simulink model "mls_driver_nasz"  (R2023a)
settings: Solver=ode5  StartTime=0.0  StopTime=inf  FixedStep=0.001  RelTol=1e-3  AbsTol=1e-6
InitFcn:
  | load ml_sensor
undefined symbols (not defined in the file or in its folder): RTDAC4PCIBaseAddress
settings Model: SimulationMode=external  ExtModeEnableFloating=off  ExtModeTrigDuration=40000  ExtModeTrigDirection=either  ExtModeArchiveFileName=exp01.mat  ExtModeArchiveDirName=h:\temp  ExtModeWriteAllDataToWs=on  Creator=Adam Pilat  LastModifiedBy=HP
settings SolverCC: AutoScaleAbsTol=off  AlgebraicLoopSolver=TrustRegion
settings DataIOCC: ExternalInput=[]  InitialState=[]  MaxDataPoints=5000  SaveFormat=Array  SignalLoggingSaveFormat=ModelDataLogs  SaveOutput=off  SaveTime=off  ReturnWorkspaceOutputs=off  SignalLoggingName=sigsOut
settings OptimizationCC: BooleanDataType=off  ExpressionDepthLimit=2147483647  InitFltsAndDblsToZero=on  LifeSpan=inf
settings DebuggingCC: SaveWithParameterizedLinksMsg=none  UnderspecifiedInitializationDetection=Classic  MergeDetectMultiDrivingBlocksExec=none  SignalResolutionControl=TryResolveAllWithWarning  MultiTaskDSMMsg=warning  MultiTaskCondExecSysMsg=none  IntegerOverflowMsg=none  FcnCallInpInsideContextMsg=warning  UnconnectedInputMsg=warning  UnconnectedOutputMsg=warning  UnconnectedLineMsg=warning  StateNameClashWarn=warning  SFUnexpectedBacktrackingDiag=warning  SFNoUnconditionalDefaultTransitionDiag=warning  SFExecutionAtInitializationDiag=none  IntegerSaturationMsg=none  ArithmeticOperatorsInVariantConditions=warning
settings HardwareCC: ProdBitPerLong=64  ProdLargestAtomicFloat=None  ProdHWDeviceType=Intel->x86-64  TargetBitPerLong=64  TargetBitPerPointer=64  TargetIntDivRoundTo=Zero  TargetEndianess=LittleEndian  TargetWordSize=64  TargetHWDeviceType=Intel->x86-64
settings ModelReferenceCC: PropagateSignalLabelsOutOfModel=off
settings SFSimCC: SimUseLocalCustomCode=off  CustomCodeUndefinedFunction=UseInterfaceOnly
settings RTWCC: Description=Real-Time Windows Target  SystemTargetFile=rtwin.tlc  TemplateMakefile=rtwin.tmf  RTWUseLocalCustomCode=off
settings CodeAppCC: StateflowObjectComments=on
settings RTWinTargetCC: TargetFcnLib=ansi_tfl_tmw.mat  TargetPreCompLibLocation=C:\Program Files\MATLAB\R2015aSP1\toolbox\sldrt\lib\win64  MultiwordTypeDef=System defined  DynamicStringBufferSize=256  ModelReferenceCompliant=off  CompOptLevelCompliant=off  GroupInternalDataByFunction=off  RemoveDisableFunc=off  RemoveResetFunc=off  MDXCompliant=off  UseToolchainInfoCompliant=off  CoderGroups=[]  AccessMethods=[]  LookupTableObjectStructAxisOrder=1,2,3,4,...  LUTObjectStructOrderExplicitValues=Size,Breakpoints,Table  LUTObjectStructOrderEvenSpacing=Size,Breakpoints,Table  ArrayLayout=Column-major  UnsupportedSFcnMsg=error  ERTHeaderFileRootName=$R$E  ERTSourceFileRootName=$R$E  ERTDataFileRootName=$R_data  OptimizeReductions=off
settings ConfigComp: CovMetricSettings=dw  CovSaveCumulativeToWorkspaceVar=on  CovSaveSingleToWorkspaceVar=on  CovExternalEMLEnable=off  CovSFcnEnable=off

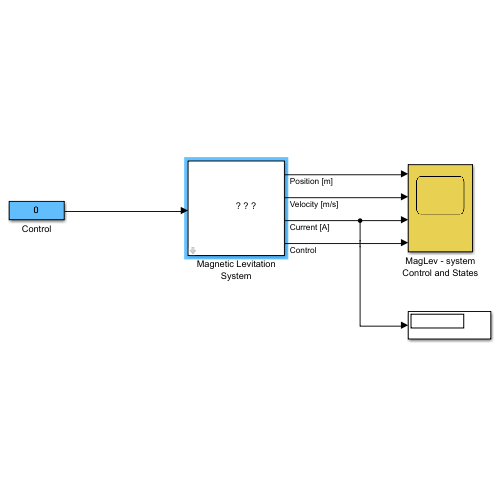
[thumbnail: Simulink's stored preview of the top-level diagram]
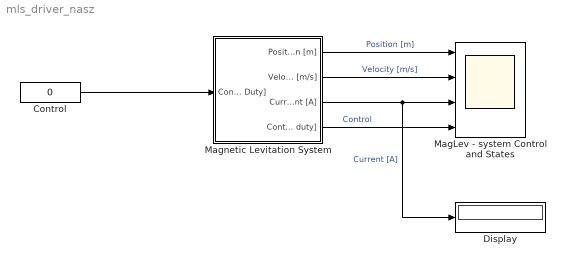
== system mls_driver_nasz ==
  Control : Constant  Value=0
  Display : Display
  MagLev - system Control and States : Scope  NumInputPorts=4
  Magnetic Levitation System : Subsystem  mask(Magnetic Levitation 1 - System){BA=RTDAC4PCIBaseAddress, T0=0.001}
      mask prompts: BA "Base Address (dec):"; T0 "Sampling period [s]:"
      mask help:
      | MagLev1 - System connection for the real-time operating mode
      | (c) InTeCo 2005
      mask Display: image(imread('MagLev1.tif'))
  wires:
  Magnetic Levitation System/1(Position [m]) -> MagLev - system Control and States/1  "Position [m]"
  Magnetic Levitation System/2(Velocity [m/s]) -> MagLev - system Control and States/2  "Velocity [m/s]"
  Magnetic Levitation System/3(Current [A]) -> Display/1, MagLev - system Control and States/3  "Current [A]"
  Magnetic Levitation System/4(Control [PWM duty]) -> MagLev - system Control and States/4  "Control"
  Control/1 -> Magnetic Levitation System/1(Control [PWM Duty])

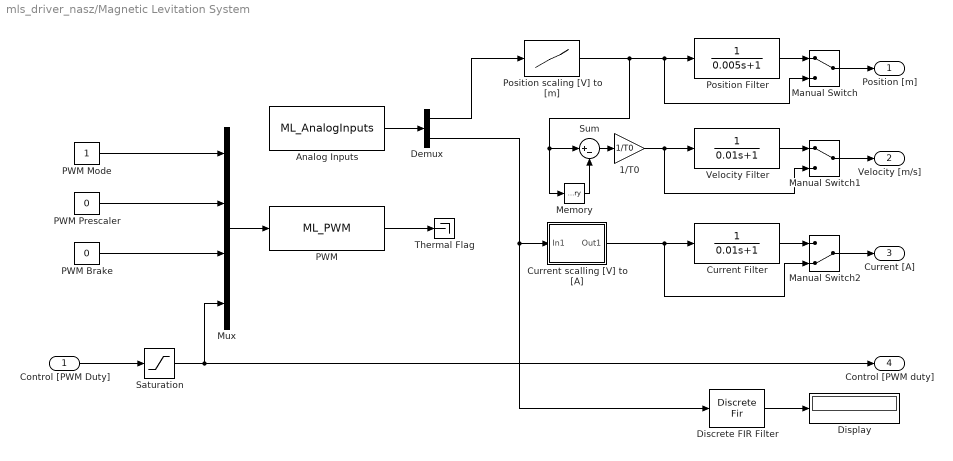
== system mls_driver_nasz/Magnetic Levitation System ==
  Control [PWM Duty] : Inport
  1/T0 : Gain  Gain=1/T0  SaturateOnIntegerOverflow=on  OutDataTypeStr=Inherit: Same as input  ParamDataTypeStr=Inherit: Same as input
  Analog Inputs : S-Function  FunctionName=ML_AnalogInputs  Parameters=BA, [4 2], [1 1], T0  SFunctionDeploymentMode=off  EnableBusSupport=off
  Current Filter : TransferFcn  Denominator=[0.01 1]
  Current scalling [V] to [A] : Subsystem
      mask Display: plot([0    0.5000    1.0000    1.5000    2.0000    2.5000], [-0.0317    0.4951    1.0302    1.5738    2.1258    2.6863]);
  Demux : Demux  Outputs=2
      settings: DisplayOption=none
  Discrete FIR Filter : DiscreteFir  Coefficients=ones(1,1000)/1000
  Display : Display
  Manual Switch : ManualSwitch
  Manual Switch1 : ManualSwitch
  Manual Switch2 : ManualSwitch  CurrentSetting=0
  Memory : Memory
  Mux : Mux
  PWM : S-Function  FunctionName=ML_PWM  Parameters=BA, T0  SFunctionDeploymentMode=off  EnableBusSupport=off
  PWM Brake : Constant  Value=0
  PWM Mode : Constant
  PWM Prescaler : Constant  Value=0
  Position Filter : TransferFcn  Denominator=[0.005 1]
  Position scaling [V] to [m] : Lookup  InputValues=SensorData.Sensor_V(end:-1:1)  Table=SensorData.Distance_m(end:-1:1)
  Saturation : Saturate  UpperLimit=1  LowerLimit=0
  Sum : Sum  Inputs=|+-  InputSameDT=on  SaturateOnIntegerOverflow=on  OutDataTypeStr=Inherit: Same as first input
  Thermal Flag : Terminator
  Velocity Filter : TransferFcn  Denominator=[0.01 1]
  Position [m] : Outport
  Velocity [m/s] : Outport  Port=2
  Current [A] : Outport  Port=3
  Control [PWM duty] : Outport  Port=4
  wires:
  Manual Switch1/1 -> Velocity [m/s]/1
  Current Filter/1 -> Manual Switch2/1
  Velocity Filter/1 -> Manual Switch1/1
  Position Filter/1 -> Manual Switch/1
  Demux/1 -> Position scaling [V] to [m]/1
  Demux/2 -> Discrete FIR Filter/1, Current scalling [V] to [A]/1(In1)
  Current scalling [V] to [A]/1(Out1) -> Manual Switch2/2, Current Filter/1
  1/T0/1 -> Manual Switch1/2, Velocity Filter/1
  Sum/1 -> 1/T0/1
  Memory/1 -> Sum/2
  Analog Inputs/1 -> Demux/1
  Mux/1 -> PWM/1
  PWM Prescaler/1 -> Mux/2
  PWM Mode/1 -> Mux/1
  PWM/1 -> Thermal Flag/1
  Saturation/1 -> Mux/4, Control [PWM duty]/1
  Control [PWM Duty]/1 -> Saturation/1
  Manual Switch2/1 -> Current [A]/1
  PWM Brake/1 -> Mux/3
  Position scaling [V] to [m]/1 -> Manual Switch/2, Position Filter/1, Memory/1, Sum/1
  Manual Switch/1 -> Position [m]/1
  Discrete FIR Filter/1 -> Display/1

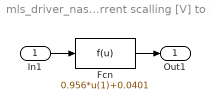
== system mls_driver_nasz/Magnetic Levitation System/Current scalling [V] to [A] ==
  In1 : Inport
  Fcn : Fcn  Expr=0.956*u(1)+0.0401
  Out1 : Outport
  wires:
  In1/1 -> Fcn/1
  Fcn/1 -> Out1/1
